simulink subsystem "pitchYawOuterLoop"  (R2026a)
settings: Solver=VariableStepAuto
values from neighbouring files (symbols this model uses):
  outerLoopParams = 0.5    [controllerParams.sldd]
settings Model: DataDictionary=controllerParams.sldd  EnableAccessToBaseWorkspace=off  Creator=maxhu  LastModifiedBy=maxhu

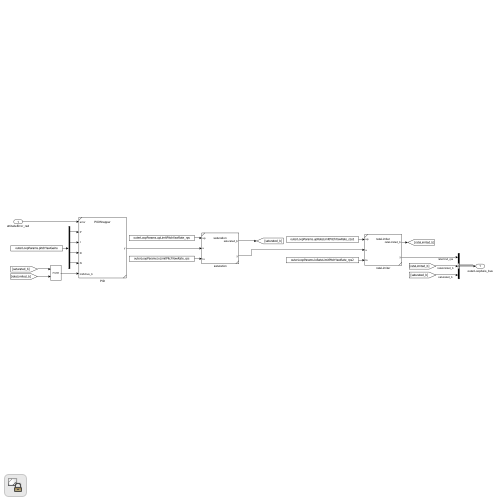
[thumbnail: Simulink's stored preview of the top-level diagram]
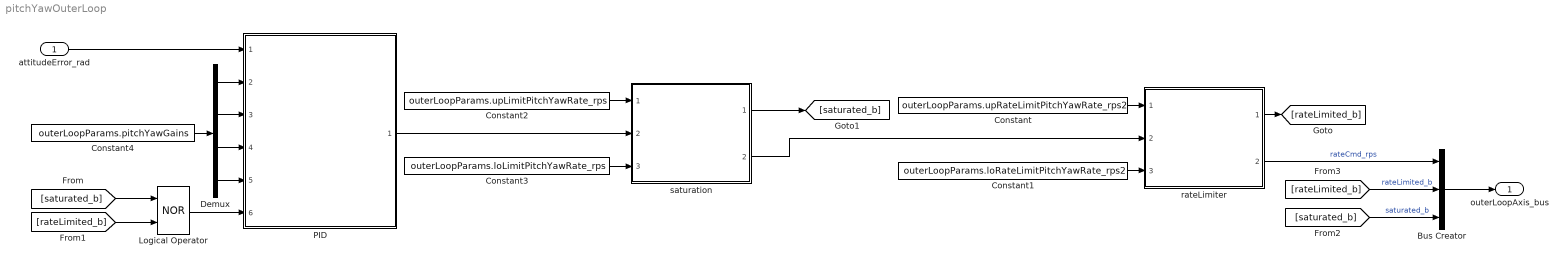
== system pitchYawOuterLoop ==
  attitudeError_rad : Inport
  Bus Creator : BusCreator  Inputs=3
  Constant : Constant  Value=outerLoopParams.upRateLimitPitchYawRate_rps2
  Constant1 : Constant  Value=outerLoopParams.loRateLimitPitchYawRate_rps2
  Constant2 : Constant  Value=outerLoopParams.upLimitPitchYawRate_rps
  Constant3 : Constant  Value=outerLoopParams.loLimitPitchYawRate_rps
  Constant4 : Constant  Value=outerLoopParams.pitchYawGains
  Demux : Demux
  Logical Operator : Logic  Operator=NOR  AllPortsSameDT=off  OutDataTypeStr=boolean
  PID : Subsystem  ReferencedSubsystem=PIDWrapper
  rateLimiter : Subsystem  ReferencedSubsystem=rateLimiter
  saturation : Subsystem  ReferencedSubsystem=saturation
  outerLoopAxis_bus : Outport
  wires:
  saturation/1 -> [saturated_b]
  Logical Operator/1 -> PID/6
  Constant3/1 -> saturation/3
  attitudeError_rad/1 -> PID/1
  Constant1/1 -> rateLimiter/3
  Constant/1 -> rateLimiter/1
  Constant2/1 -> saturation/1
  [saturated_b] -> Logical Operator/1
  Demux/1 -> PID/2
  Demux/4 -> PID/5
  Demux/3 -> PID/4
  Demux/2 -> PID/3
  Constant4/1 -> Demux/1
  [saturated_b] -> Bus Creator/3  "saturated_b"
  [rateLimited_b] -> Bus Creator/2  "rateLimited_b"
  Bus Creator/1 -> outerLoopAxis_bus/1
  PID/1 -> saturation/2
  saturation/2 -> rateLimiter/2
  [rateLimited_b] -> Logical Operator/2
  rateLimiter/1 -> [rateLimited_b]
  rateLimiter/2 -> Bus Creator/1  "rateCmd_rps"
